simulink model "tadpole_dynamic_close_loop"  (R2019b)
settings: Solver=FixedStepAuto  StartTime=0.0  StopTime=sim_time  FixedStep=0.001  RelTol=1e-2
values from neighbouring files (symbols this model uses):
  C_alpha = 1000*ones(runcycle,1)    [rand_par.m]    (also in whole_par.m = 1000; whole_par_bias.m = 1000)
  C_beta = 50*ones(runcycle,1)    [rand_par.m]    (also in whole_par.m = 50; whole_par_bias.m = 50)
  Cd = 0.25*ones(runcycle,1)    [rand_par.m]    (also in whole_par.m = 0.25; whole_par_bias.m = 0.25)
  delta_fL = -1*ones(runcycle,1)    [rand_par.m]    (also in whole_par.m = -1; whole_par_bias.m = -1)
  delta_fR = 3.5*ones(runcycle,1)    [rand_par.m]    (also in whole_par.m = 3.5; whole_par_bias.m = 3.5)
  FA = 1*ones(runcycle,1)    [rand_par.m]    (also in whole_par.m = 1; whole_par_bias.m = 1)
  h = [ h(1:j-1) ; h(j+1:m)]    [UMDIRECT.m]    (also in whole_par.m = 0.4896; whole_par_bias.m = 0.4896)
  I_f_wheel = 0.3    [whole_par.m]    (also in whole_par_bias.m)
  I_r_wheel = 0.5    [whole_par.m]    (also in whole_par_bias.m)
  I_x = 12.1*ones(runcycle,1)    [rand_par.m]    (also in whole_par.m = 12.1; whole_par_bias.m = 12.1)
  I_y = 36.7*ones(runcycle,1)    [rand_par.m]    (also in whole_par.m = 36.7; whole_par_bias.m = 36.7)
  I_z = 50*DOE(:,2)    [rand_par.m]    (also in whole_par.m = 50; whole_par_bias.m = 60)
  k_z = 30000*ones(runcycle,1)    [rand_par.m]    (also in whole_par.m = 30000; whole_par_bias.m = 30000)
  l_1 = 0.724    [whole_par.m]    (also in whole_par_bias.m)
  l_2 = 0.719    [whole_par.m]    (also in whole_par_bias.m)
  m = m - 1    [UMDIRECT.m]    (also in rand_par.m = 48.3*DOE(:,1); whole_par.m = 48.3; whole_par_bias.m = 60)
  mu_dp = 0.8*ones(runcycle,1)    [rand_par.m]    (also in whole_par.m = 0.8; whole_par_bias.m = 0.8)
  mu_lp = 0.8*ones(runcycle,1)    [rand_par.m]    (also in whole_par.m = 0.8; whole_par_bias.m = 0.8)
  mu_rolling_1 = 0.009*ones(runcycle,1)    [rand_par.m]    (also in whole_par.m = 0.009; whole_par_bias.m = 0.009)
  mu_rolling_2 = 0.0005*ones(runcycle,1)    [rand_par.m]    (also in whole_par.m = 0.0005; whole_par_bias.m = 0.0005)
  R_0 = 0.335*ones(runcycle,1)    [rand_par.m]    (also in whole_par.m = 0.335; whole_par_bias.m = 0.335)
  rho = 1.225*ones(runcycle,1)    [rand_par.m]    (also in whole_par.m = 1.225; whole_par_bias.m = 1.225)
  SAP = 0.01*ones(runcycle,1)    [rand_par.m]    (also in whole_par.m = 0.01; whole_par_bias.m = 0.01)
  V_wind = 0*ones(runcycle,1)    [rand_par.m]    (also in whole_par.m = 0; whole_par_bias.m = 0)
  waypoint = [x' y']    [waypoints.m]
undefined symbols (not defined in the file or in its folder): DiscIntNeverNeededParam
libraries: simulink_extras x11, simulink x2, robotalgslib x1, mobileRoboticsLib x1
(part 2 of 4)

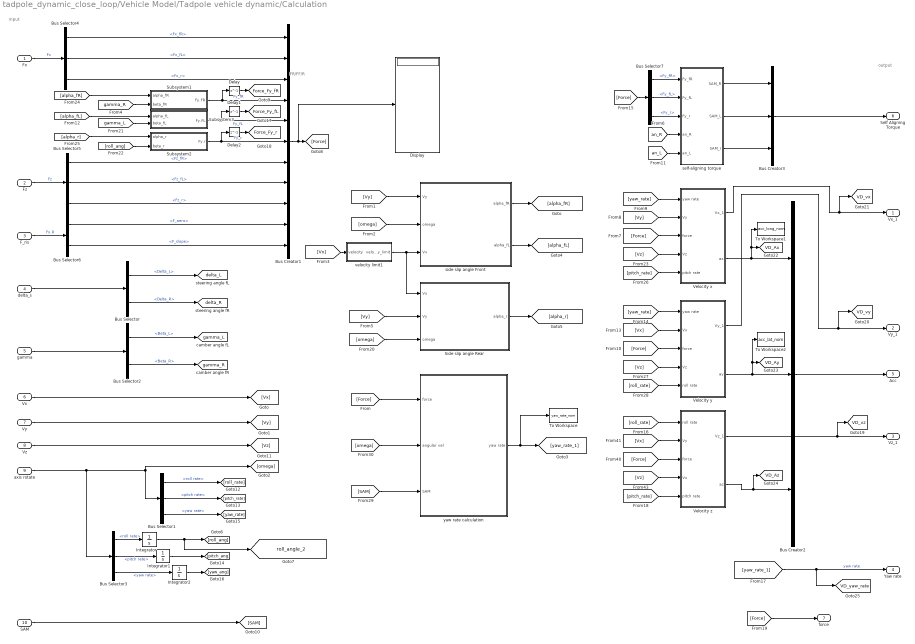
== system tadpole_dynamic_close_loop/Vehicle Model/Tadpole vehicle dynamic/Calculation ==
  note: input
  note: output
  note: FR/FF/R
  Fx : Inport
  Fz : Inport  Port=2
  F_ris : Inport  Port=3
  delta_s : Inport  Port=4
  gamma : Inport  Port=5
  Vx : Inport  Port=6
  Vy : Inport  Port=7
  Vz : Inport  Port=8
  axis rotate : Inport  Port=9
  SAM : Inport  Port=10
  Bus Creator1 : BusCreator  Inputs=11
  Bus Creator2 : BusCreator  Inputs=3
  Bus Creator3 : BusCreator  Inputs=3
  Bus Selector : BusSelector  OutputSignals=Delta_L,Delta_R
  Bus Selector1 : BusSelector  OutputSignals=roll rate,pitch rate,yaw rate
  Bus Selector2 : BusSelector  OutputSignals=Beta_L,Beta_R
  Bus Selector3 : BusSelector  OutputSignals=roll rate,pitch rate,yaw rate
  Bus Selector4 : BusSelector  OutputSignals=Fx_fR,Fx_fL,Fx_r
  Bus Selector5 : BusSelector  OutputSignals=Fz_fR,Fz_fL,Fz_r
  Bus Selector6 : BusSelector  OutputSignals=F_aero,F_slope
  Bus Selector7 : BusSelector  OutputSignals=Fy_fR,Fy_fL,Fy_r
  Delay : Delay  DelayLength=1
  Delay1 : Delay  DelayLength=1
  Delay2 : Delay  DelayLength=1
  Display : Display
  Integrator : Integrator
  Integrator1 : Integrator
  Integrator2 : Integrator
  Side slip angle Rear : Subsystem
  Subsystem1 : Subsystem
  Subsystem2 : Subsystem
  Subsystem3 : Subsystem
  To Workspace : ToWorkspace  VariableName=yaw_rate_nom  SaveFormat=Timeseries  SampleTime=-1
  To Workspace1 : ToWorkspace  VariableName=acc_long_nom  SaveFormat=Timeseries  SampleTime=-1
  To Workspace2 : ToWorkspace  VariableName=acc_lat_nom  SaveFormat=Timeseries  SampleTime=-1
  Velocity x : Subsystem
  Velocity y : Subsystem
  Velocity z : Subsystem
  self-aligning torque : Subsystem
  side slip angle Front : Subsystem
  velocity limit1 : Subsystem
  yaw rate calculation : Subsystem
  Vx_1 : Outport  VectorParamsAs1DForOutWhenUnconnected=off
  Vy_1 : Outport  Port=2  VectorParamsAs1DForOutWhenUnconnected=off
  Vz_1 : Outport  Port=3  VectorParamsAs1DForOutWhenUnconnected=off
  Yaw rate : Outport  Port=4  VectorParamsAs1DForOutWhenUnconnected=off
  Acc : Outport  Port=5  VectorParamsAs1DForOutWhenUnconnected=off
  Self Aligning Torque : Outport  Port=6  VectorParamsAs1DForOutWhenUnconnected=off
  force : Outport  Port=7  VectorParamsAs1DForOutWhenUnconnected=off
  tag scope: Force_Fy_fL=global, Force_Fy_fR=global, Force_Fy_r=global, VD_Ax=global, VD_Ay=global, VD_Az=global, VD_vx=global, VD_vy=global, VD_vz=global, VD_yaw_rate=global, delta_L=global, delta_R=global, gamma_L=global, gamma_R=global, roll_angle_2=global
  wires:
  delta_s/1 -> Bus Selector/1
  Bus Selector/1 -> [delta_L]  "<Delta_L>"
  Bus Selector/2 -> [delta_R]  "<Delta_R>"
  Vx/1 -> [Vx]
  Vy/1 -> [Vy]
  [Force] -> yaw rate calculation/1(force)
  yaw rate calculation/1(yaw rate) -> To Workspace/1, [yaw_rate_1]
  Bus Creator1/1 -> Display/1, [Force]
  [Vy] -> side slip angle Front/1(Vy)
  [omega] -> side slip angle Front/2(omega)
  [omega] -> Side slip angle Rear/3(omega)
  [Vy] -> Side slip angle Rear/2(Vy)
  side slip angle Front/1(alpha_fR) -> [alpha_fR]
  side slip angle Front/2(alpha_fL) -> [alpha_fL]
  Side slip angle Rear/1(alpha_r) -> [alpha_r]
  self-aligning torque/1(SAM_R) -> Bus Creator3/1
  self-aligning torque/2(SAM_L) -> Bus Creator3/2
  [Vx] -> velocity limit1/1("velocity ")
  velocity limit1/1("velocity_limit ") -> Side slip angle Rear/1(Vx), side slip angle Front/3(Vx)
  [yaw_rate] -> Velocity x/1(yaw rate)
  [Vy] -> Velocity x/2(Vy)
  [Force] -> Velocity x/3("force ")
  Velocity x/1(Vx_1) -> [VD_vx], Vx_1/1
  Velocity x/2(ax) -> To Workspace1/1, [VD_Ax], Bus Creator2/1
  [Force] -> Velocity y/3("force ")
  Velocity y/1(Vy_1) -> [VD_vy], Vy_1/1
  [yaw_rate] -> Velocity y/1(yaw rate)
  [Vx] -> Velocity y/2(Vx)
  Velocity y/2(ay) -> To Workspace2/1, [VD_Ay], Bus Creator2/2
  [yaw_rate_1] -> [VD_yaw_rate], Yaw rate/1  "yaw rate"
  SAM/1 -> [SAM]
  [Vz] -> Velocity x/4(Vz)
  [pitch_rate] -> Velocity x/5(pitch rate)
  Vz/1 -> [Vz]
  Bus Selector1/1 -> [roll_rate]  "<roll rate>"
  Bus Selector1/2 -> [pitch_rate]  "<pitch rate>"
  Bus Selector1/3 -> [yaw_rate]  "<yaw rate>"
  [Vz] -> Velocity y/4(Vz)
  [roll_rate] -> Velocity y/5(roll rate)
  [SAM] -> yaw rate calculation/3(SAM)
  [omega] -> yaw rate calculation/2(angular vel)
  self-aligning torque/3(SAM_r) -> Bus Creator3/3
  Velocity z/1(Vz_1) -> [VD_vz], Vz_1/1
  [Vx] -> Velocity z/2(Vy)
  [pitch_rate] -> Velocity z/5(pitch rate)
  [roll_rate] -> Velocity z/1(roll rate)
  [Force] -> Velocity z/3("force ")
  Velocity z/2(az) -> [VD_Az], Bus Creator2/3
  [Vz] -> Velocity z/4(Vx)
  Bus Creator2/1 -> Acc/1
  Bus Creator3/1 -> Self Aligning Torque/1
  gamma/1 -> Bus Selector2/1
  Bus Selector2/1 -> [gamma_L]  "<Beta_L>"
  Bus Selector2/2 -> [gamma_R]  "<Beta_R>"
  Bus Selector3/3 -> Integrator2/1  "<yaw rate>"
  Bus Selector3/2 -> Integrator1/1  "<pitch rate>"
  Bus Selector3/1 -> Integrator/1  "<roll rate>"
  axis rotate/1 -> Bus Selector3/1, [omega], Bus Selector1/1
  Integrator/1 -> [roll_angle_2], [roll_ang]
  Integrator1/1 -> [pitch_ang]
  Integrator2/1 -> [yaw_ang]
  Fx/1 -> Bus Selector4/1  "Fx"
  Bus Selector4/1 -> Bus Creator1/1  "<Fx_fR>"
  Bus Selector4/2 -> Bus Creator1/2  "<Fx_fL>"
  Bus Selector4/3 -> Bus Creator1/3  "<Fx_r>"
  [gamma_L] -> Subsystem3/2(beta_fL)
  [alpha_fR] -> Subsystem1/1(alpha_fR)
  [gamma_R] -> Subsystem1/2(beta_fR)
  [alpha_fL] -> Subsystem3/1(alpha_fL)
  [roll_ang] -> Subsystem2/2(beta_r)
  [alpha_r] -> Subsystem2/1(alpha_r)
  Subsystem1/1(Fy.FR) -> Bus Creator1/4, Delay/1  "Fy_fR"
  Subsystem3/1(Fy.FL) -> Delay1/1, Bus Creator1/5  "Fy_fL"
  Subsystem2/1(Fy.r) -> Delay2/1, Bus Creator1/6  "Fy_r"
  Fz/1 -> Bus Selector5/1  "Fz"
  Bus Selector5/2 -> Bus Creator1/8  "<Fz_fL>"
  Bus Selector5/1 -> Bus Creator1/7  "<Fz_fR>"
  Bus Selector5/3 -> Bus Creator1/9  "<Fz_r>"
  F_ris/1 -> Bus Selector6/1  "Fx.R"
  Bus Selector6/1 -> Bus Creator1/10  "<F_aero>"
  Bus Selector6/2 -> Bus Creator1/11  "<F_slope>"
  [Force] -> force/1
  [an_R] -> self-aligning torque/4(an_R)
  [an_L] -> self-aligning torque/5(an_L)
  [Force] -> Bus Selector7/1
  Bus Selector7/1 -> self-aligning torque/1(Fy_fR)  "<Fy_fR>"
  Bus Selector7/2 -> self-aligning torque/2(Fy_fL)  "<Fy_fL>"
  Bus Selector7/3 -> self-aligning torque/3(Fy_r)  "<Fy_r>"
  Delay/1 -> [Force_Fy_fR]
  Delay1/1 -> [Force_Fy_fL]
  Delay2/1 -> [Force_Fy_r]

== system tadpole_dynamic_close_loop/Vehicle Model/Tadpole vehicle dynamic/Velocity ==
  Vx : Inport
  Vy : Inport  Port=2
  Add : Sum
  Power : Math  Operator=pow  SaturateOnIntegerOverflow=on
  Power1 : Math  Operator=pow  SaturateOnIntegerOverflow=on
  Sqrt : Sqrt  SaturateOnIntegerOverflow=on
  power : Constant  Value=2
  power 2 : Constant  Value=2
  absolute V : Outport  VectorParamsAs1DForOutWhenUnconnected=off
  wires:
  Power1/1 -> Add/2  "Vy^2"
  power/1 -> Power1/2
  Power/1 -> Add/1  "Vx^2"
  power 2/1 -> Power/2
  Vx/1 -> Power/1
  Vy/1 -> Power1/1
  Add/1 -> Sqrt/1
  Sqrt/1 -> absolute V/1

== system tadpole_dynamic_close_loop/Vehicle Model/Tadpole vehicle dynamic/local to global ==
  Vy : Inport
  yaw rate : Inport  Port=2
  Vx : Inport  Port=3
  Add : Sum
  Add1 : Sum
  Gain : Gain  Gain=-1
  Integrator : Integrator
  Multiply{,1..3} (4 alike) : Product
  Sin : Trigonometry
  Sin1 : Trigonometry  Operator=cos
  absolute x dot : Outport  VectorParamsAs1DForOutWhenUnconnected=off
  absolute y dot : Outport  Port=2  VectorParamsAs1DForOutWhenUnconnected=off
  tag scope: VD_yaw_angle=global
  wires:
  Gain/1 -> Add/2
  Vx/1 -> Multiply/2, Multiply2/2
  Multiply1/1 -> Gain/1
  Sin/1 -> Multiply2/1, Multiply1/1
  Multiply3/1 -> Add1/2
  Integrator/1 -> [VD_yaw_angle], [A]
  Sin1/1 -> Multiply3/1, Multiply/1
  Multiply/1 -> Add/1
  Vy/1 -> Multiply3/2, Multiply1/2
  Add/1 -> absolute x dot/1  "absolute x dot"
  [A] -> Sin1/1, Sin/1
  Multiply2/1 -> Add1/1
  Add1/1 -> absolute y dot/1
  yaw rate/1 -> Integrator/1

== system tadpole_dynamic_close_loop/Vehicle Model/resistance calculation/Aerodynamic Drag Force ==
  Vx : Inport
  Add : Sum
  Air density : Constant  Value=rho
  Constant : Constant  Value=V_wind
  Constant5 : Constant  Value=0.5
  Constant6 : Constant  Value=2
  "Drag coefficient " : Constant  Value=Cd
  Front Area : Constant  Value=FA
  Gain : Gain  Gain=-1
  Math Function : Math  Operator=pow  SaturateOnIntegerOverflow=on
  Product1 : Product  Inputs=6
  Sign : Signum
  F_aero : Outport  VectorParamsAs1DForOutWhenUnconnected=off
  wires:
  Add/1 -> Math Function/1, Sign/1
  Constant6/1 -> Math Function/2
  "Drag coefficient "/1 -> Product1/3
  Product1/1 -> F_aero/1
  Math Function/1 -> Product1/5
  Constant5/1 -> Product1/1
  Air density/1 -> Product1/4
  Front Area/1 -> Product1/2
  Sign/1 -> Gain/1
  Gain/1 -> Product1/6
  Vx/1 -> Add/1
  Constant/1 -> Add/2

== system tadpole_dynamic_close_loop/Vehicle Model/resistance calculation/Rear Traction add up ==
  break : Inport
  motor : Inport  Port=2
  V sign : Inport  Port=3
  Abs : Abs
  Abs1 : Abs
  Fm<0 : Subsystem  TreatAsAtomicUnit=on
  Fm>=0 : Subsystem  TreatAsAtomicUnit=on
  If (check motor sign) : If  IfExpression=u1 >= 0
  Merge : Merge
  Scope : Scope
  Rear Traction : Outport  VectorParamsAs1DForOutWhenUnconnected=off
  wires:
  Abs/1 -> Fm<0/1(|break|), Scope/1, Fm>=0/1(|break|)  "break"
  motor/1 -> If (check motor sign)/1, Abs1/1
  Abs1/1 -> Fm<0/2(|motor|), Fm>=0/2(|motor|)  "motor"
  break/1 -> Abs/1
  If (check motor sign)/1 -> Fm>=0/Action
  If (check motor sign)/2 -> Fm<0/Action
  Fm>=0/1(Out1) -> Merge/1
  Fm<0/1(Out1) -> Merge/2
  Merge/1 -> Rear Traction/1
  V sign/1 -> Fm<0/3("velocity sign "), Fm>=0/3("velocity sign ")  "velocity sign"

== system tadpole_dynamic_close_loop/Vehicle Model/resistance calculation/Rolling Resistance Force Front L ==
  Fz_fL : Inport
  Vx : Inport  Port=2
  Vy : Inport  Port=3
  yaw rate : Inport  Port=4
  Delta_L : Inport  Port=5
  Gain : Gain  Gain=-1
  Multiply : Product  Inputs=3
  Scope : Scope
  Sign : Signum
  Subsystem : Subsystem
  mu(v) : Subsystem
  Frr_fL : Outport  VectorParamsAs1DForOutWhenUnconnected=off
  wires:
  Fz_fL/1 -> Multiply/1  "Fzr"
  Subsystem/1(Vx_Wheel) -> mu(v)/1(Vx), Sign/1
  Gain/1 -> Multiply/3
  mu(v)/1(mu_rolling) -> Multiply/2
  Sign/1 -> Gain/1
  Vx/1 -> Subsystem/1(Vx)
  Vy/1 -> Subsystem/2(Vy)
  yaw rate/1 -> Subsystem/3(yaw rate)
  Delta_L/1 -> Subsystem/4(Delta_L)
  Multiply/1 -> Scope/1, Frr_fL/1

== system tadpole_dynamic_close_loop/Vehicle Model/resistance calculation/Rolling Resistance Force Front R ==
  Fz_fR : Inport
  Vx : Inport  Port=2
  Vy : Inport  Port=3
  yaw rate : Inport  Port=4
  Delta_R : Inport  Port=5
  Gain : Gain  Gain=-1
  Multiply : Product  Inputs=3
  Sign : Signum
  Subsystem : Subsystem
  mu(v) : Subsystem
  Frr_fR : Outport  VectorParamsAs1DForOutWhenUnconnected=off
  wires:
  Fz_fR/1 -> Multiply/1  "Fzr"
  Subsystem/1(Vx_Wheel) -> mu(v)/1(Vx), Sign/1
  Gain/1 -> Multiply/3
  mu(v)/1(mu_rolling) -> Multiply/2
  Sign/1 -> Gain/1
  Vx/1 -> Subsystem/1(Vx)
  Vy/1 -> Subsystem/2(Vy)
  yaw rate/1 -> Subsystem/3(yaw rate)
  Delta_R/1 -> Subsystem/4(Delta_R)
  Multiply/1 -> Frr_fR/1

== system tadpole_dynamic_close_loop/Vehicle Model/resistance calculation/Rolling Resistance Force Rear ==
  Fz_r : Inport
  velocity sign : Inport  Port=2
  Vx : Inport  Port=3
  Gain : Gain  Gain=-1
  Multiply : Product  Inputs=3
  mu(v) : Subsystem
  Frr : Outport  VectorParamsAs1DForOutWhenUnconnected=off
  wires:
  Multiply/1 -> Frr/1
  Fz_r/1 -> Multiply/1  "Fzr"
  velocity sign/1 -> Gain/1
  Gain/1 -> Multiply/3
  mu(v)/1(mu_rolling) -> Multiply/2
  Vx/1 -> mu(v)/1(Vx)

== system tadpole_dynamic_close_loop/Vehicle Model/resistance calculation/linear slip cal.  ==
  rear traction : Inport
  rear normal force : Inport  Port=2
  Display : Display
  Gain2 : Gain  Gain=-1
  MinMax : MinMax  Inputs=2
  MinMax2 : MinMax  Function=max  Inputs=2
  Product : Product
  max. long. friction coefficient : Constant  Value=mu_dp
  slip recgonition : Subsystem
  "Rear Traction " : Outport  VectorParamsAs1DForOutWhenUnconnected=off
  wires:
  Gain2/1 -> MinMax2/2
  Product/1 -> Gain2/1, slip recgonition/1(In2), MinMax/1
  MinMax/1 -> slip recgonition/2(In3), Display/1, MinMax2/1
  MinMax2/1 -> "Rear Traction "/1
  rear traction/1 -> MinMax/2
  rear normal force/1 -> Product/2
  max. long. friction coefficient/1 -> Product/1

== system tadpole_dynamic_close_loop/Vehicle Model/resistance calculation/slope  ==
  Slope : Inport
  Degrees to Radians : simulink_extras/Transformations/Degrees to Radians
  Gain : Gain  Gain=-1
  Gain1 : Gain  Gain=9.81
  Product : Product
  Sin : Trigonometry
  mass : Constant  Value=m
  F_slope : Outport  VectorParamsAs1DForOutWhenUnconnected=off
  wires:
  Gain1/1 -> Product/1
  Sin/1 -> Product/2
  Slope/1 -> Degrees to Radians/1
  Product/1 -> Gain/1  "Slope"
  Gain/1 -> F_slope/1
  mass/1 -> Gain1/1
  Degrees to Radians/1 -> Sin/1

== system tadpole_dynamic_close_loop/Vehicle Model/resistance calculation/torque to force ==
  traction torque : Inport
  rear normal force : Inport  Port=2
  Add : Sum  Inputs=+-
  Divide1 : Product  Inputs=*/
  Divide2 : Product  Inputs=*/
  Initial wheel radius : Constant  Value=R_0
  tire vertical stiffness : Constant  Value=k_z
  rear traction F : Outport  VectorParamsAs1DForOutWhenUnconnected=off
  tag scope: R_h=global
  wires:
  traction torque/1 -> Divide1/1
  Divide1/1 -> rear traction F/1
  tire vertical stiffness/1 -> Divide2/2
  rear normal force/1 -> Divide2/1
  Divide2/1 -> Add/2
  Initial wheel radius/1 -> Add/1
  Add/1 -> [R_h], Divide1/2  "effective radius"

== system tadpole_dynamic_close_loop/Vehicle Model/resistance calculation/velocity limit x ==
  "velocity " : Inport
  If Action Subsystem2 : Subsystem  TreatAsAtomicUnit=on
  If Action Subsystem3 : Subsystem  TreatAsAtomicUnit=on
  If1 : If  IfExpression=u1>0
  Merge : Merge
  "velocity_limit " : Outport  VectorParamsAs1DForOutWhenUnconnected=off
  wires:
  Merge/1 -> "velocity_limit "/1
  "velocity "/1 -> If Action Subsystem3/1(In1), If Action Subsystem2/1(In1), If1/1
  If1/1 -> If Action Subsystem2/Action
  If1/2 -> If Action Subsystem3/Action
  If Action Subsystem2/1(Out1) -> Merge/1
  If Action Subsystem3/1(Out1) -> Merge/2

== system tadpole_dynamic_close_loop/Vehicle Model/resistance calculation/velocity limit y ==
  "velocity " : Inport
  If Action Subsystem2 : Subsystem  TreatAsAtomicUnit=on
  If Action Subsystem3 : Subsystem  TreatAsAtomicUnit=on
  If1 : If  IfExpression=u1>0
  Merge : Merge
  "velocity_limit " : Outport  VectorParamsAs1DForOutWhenUnconnected=off
  wires:
  Merge/1 -> "velocity_limit "/1
  "velocity "/1 -> If Action Subsystem3/1(In1), If Action Subsystem2/1(In1), If1/1
  If1/1 -> If Action Subsystem2/Action
  If1/2 -> If Action Subsystem3/Action
  If Action Subsystem2/1(Out1) -> Merge/1
  If Action Subsystem3/1(Out1) -> Merge/2

== system tadpole_dynamic_close_loop/Vehicle Model/Tadpole vehicle dynamic/Calculation/Side slip angle Rear ==
  Vx : Inport
  Vy : Inport  Port=2
  omega : Inport  Port=3
  Add : Sum  Inputs=+-
  Atan1 : Trigonometry  Operator=atan
  Bus Selector : BusSelector  OutputSignals=yaw rate
  Constant : Constant
  Constant1 : Constant
  Constant4 : Constant  Value=0
  Constant7 : Constant  Value=l_2
  Divide4 : Product  Inputs=*/
  Minus1 : Sum  Inputs=+-
  Multiply1 : Product
  Product : Product
  Radians to Degrees1 : simulink_extras/Transformations/Radians to Degrees
  Switch : Switch  Criteria=u2 ~= 0
  Switch1 : Switch  Criteria=u2 ~= 0
  delta_rear : Constant  Value=0
  velocity limit1 : Subsystem
  alpha_r : Outport  VectorParamsAs1DForOutWhenUnconnected=off
  tag scope: VD_Vy_r=global, VD_alpha_r=global
  wires:
  Switch/1 -> Divide4/2
  Constant/1 -> Switch/3
  Divide4/1 -> Atan1/1
  Add/1 -> Product/1  "alpha_r"
  Constant7/1 -> Multiply1/1
  Vy/1 -> Minus1/1
  Atan1/1 -> Add/2
  Minus1/1 -> [VD_Vy_r], Divide4/1
  Multiply1/1 -> Minus1/2
  [yaw_rate] -> Multiply1/2
  omega/1 -> Bus Selector/1
  Bus Selector/1 -> [yaw_rate]  "<yaw rate>"
  delta_rear/1 -> Add/1
  Constant4/1 -> Switch1/3
  Vx/1 -> velocity limit1/1("velocity "), Switch/1, Switch/2
  Switch1/1 -> Product/2
  Constant1/1 -> Switch1/1
  velocity limit1/1("velocity_limit ") -> Switch1/2
  Product/1 -> Radians to Degrees1/1, alpha_r/1
  Radians to Degrees1/1 -> [VD_alpha_r]

== system tadpole_dynamic_close_loop/Vehicle Model/Tadpole vehicle dynamic/Calculation/Subsystem1 ==
  alpha_fR : Inport
  beta_fR : Inport  Port=2
  Add : Sum
  Bus Selector : BusSelector  OutputSignals=Vx
  Gain : Gain  Gain=C_alpha
  Gain1 : Gain  Gain=C_beta
  IC : InitialCondition  Value=0
  Product : Product
  Scope : Scope  NumInputPorts=3
  Sign : Signum
  Subsystem : Subsystem
  velocity limit : Subsystem
  Fy.FR : Outport  VectorParamsAs1DForOutWhenUnconnected=off
  tag scope: Force_Fy_fR_camber=global, Force_Fy_fR_sideslip=global
  wires:
  Gain/1 -> [Force_Fy_fR_sideslip], Scope/1, Add/1  "Fy.FR sideslip"
  alpha_fR/1 -> Gain/1
  Add/1 -> Product/1
  Gain1/1 -> [Force_Fy_fR_camber], Scope/2, Add/2  "Fy.FR camber"
  beta_fR/1 -> Gain1/1
  [V] -> Bus Selector/1
  velocity limit/1("velocity_limit ") -> Sign/1
  Sign/1 -> Scope/3, Product/2
  Product/1 -> Subsystem/1(Fy_fR)
  Bus Selector/1 -> velocity limit/1("velocity ")  "<Vx>"
  Subsystem/1(Lateral force fR) -> IC/1
  IC/1 -> Fy.FR/1

== system tadpole_dynamic_close_loop/Vehicle Model/Tadpole vehicle dynamic/Calculation/Subsystem2 ==
  alpha_r : Inport
  beta_r : Inport  Port=2
  Add : Sum
  Bus Selector : BusSelector  OutputSignals=Vx
  Gain2 : Gain  Gain=C_alpha
  Gain3 : Gain  Gain=C_beta
  Product : Product
  Sign : Signum
  Subsystem : Subsystem
  velocity limit : Subsystem
  Fy.r : Outport  VectorParamsAs1DForOutWhenUnconnected=off
  tag scope: Force_Fy_r_camber=global, Force_Fy_r_sideslip=global
  wires:
  beta_r/1 -> Gain3/1
  Gain3/1 -> [Force_Fy_r_camber], Add/2  "Fy.r camber"
  alpha_r/1 -> Gain2/1
  Add/1 -> Product/1
  Gain2/1 -> [Force_Fy_r_sideslip], Add/1  "Fy.r sideslip"
  velocity limit/1("velocity_limit ") -> Sign/1
  Sign/1 -> Product/2
  Product/1 -> Subsystem/1(Fy_fL)
  [V] -> Bus Selector/1
  Bus Selector/1 -> velocity limit/1("velocity ")  "<Vx>"
  Subsystem/1(Lateral Force r) -> Fy.r/1

== system tadpole_dynamic_close_loop/Vehicle Model/Tadpole vehicle dynamic/Calculation/Subsystem3 ==
  alpha_fL : Inport
  beta_fL : Inport  Port=2
  Add : Sum
  Bus Selector : BusSelector  OutputSignals=Vx
  Gain1 : Gain  Gain=C_alpha
  Gain2 : Gain  Gain=C_beta
  Product : Product
  Sign : Signum
  Subsystem : Subsystem
  velocity limit : Subsystem
  Fy.FL : Outport  VectorParamsAs1DForOutWhenUnconnected=off
  tag scope: Force_Fy_fL_camber=global, Force_Fy_fL_sideslip=global
  wires:
  Add/1 -> Product/1
  alpha_fL/1 -> Gain1/1
  beta_fL/1 -> Gain2/1
  Gain1/1 -> [Force_Fy_fL_sideslip], Add/1  "Fy.FL sideslip"
  Gain2/1 -> [Force_Fy_fL_camber], Add/2  "Fy.FL camber"
  velocity limit/1("velocity_limit ") -> Sign/1
  Sign/1 -> Product/2
  Product/1 -> Subsystem/1(Fy_fL)
  [V] -> Bus Selector/1
  Bus Selector/1 -> velocity limit/1("velocity ")  "<Vx>"
  Subsystem/1(Lateral Force fL) -> Fy.FL/1

== system tadpole_dynamic_close_loop/Vehicle Model/Tadpole vehicle dynamic/Calculation/Velocity x ==
  note: Vx'
  note: Equation of Vx
  note: Vx
  yaw rate : Inport
  Vy : Inport  Port=2
  "force " : Inport  Port=3
  Vz : Inport  Port=4
  pitch rate : Inport  Port=5
  Add : Sum  Inputs=-++
  Bus Selector : BusSelector  OutputSignals=Fx_fR,Fx_fL,Fy_fR,Fy_fL,Fx_r
  Divide : Product  Inputs=*/
  Equivalent mass : Subsystem
  Gain : Gain  Gain=-1
  Gain1 : Gain  Gain=-1
  Integrator : Integrator
  Multiply{1..4} (4 alike) : Product
  Product : Product
  Product1 : Product
  Sin1 : Trigonometry  Operator=cos
  Sin2 : Trigonometry  Operator=cos
  Sin3 : Trigonometry
  Sin4 : Trigonometry
  Sum1 : Sum  Inputs=+++++
  Vx_1 : Outport  VectorParamsAs1DForOutWhenUnconnected=off
  ax : Outport  Port=2  VectorParamsAs1DForOutWhenUnconnected=off
  tag scope: Force_Fx=global
  wires:
  Product/1 -> Add/2
  yaw rate/1 -> Product/2
  Vy/1 -> Product/1
  Integrator/1 -> Vx_1/1
  Add/1 -> ax/1, Integrator/1
  "force "/1 -> Bus Selector/1
  Bus Selector/1 -> Multiply2/2  "<Fx_fR>"
  Sin2/1 -> Multiply2/1
  [delta_R] -> Sin2/1
  Sin1/1 -> Multiply1/1
  [delta_L] -> Sin1/1
  Bus Selector/2 -> Multiply1/2  "<Fx_fL>"
  [delta_R] -> Sin3/1
  Sin3/1 -> Multiply3/1
  Bus Selector/3 -> Gain/1  "<Fy_fR>"
  Gain/1 -> Multiply3/2
  Sin4/1 -> Multiply4/1
  [delta_L] -> Sin4/1
  Gain1/1 -> Multiply4/2
  Bus Selector/4 -> Gain1/1  "<Fy_fL>"
  Multiply2/1 -> Sum1/1
  Multiply1/1 -> Sum1/2
  Multiply3/1 -> Sum1/3
  Multiply4/1 -> Sum1/4
  Bus Selector/5 -> Sum1/5  "<Fx_r>"
  Sum1/1 -> [Force_Fx], Divide/1
  Divide/1 -> Add/3
  Vz/1 -> Product1/1
  pitch rate/1 -> Product1/2
  Product1/1 -> Add/1
  Equivalent mass/1(Mass_eq) -> Divide/2

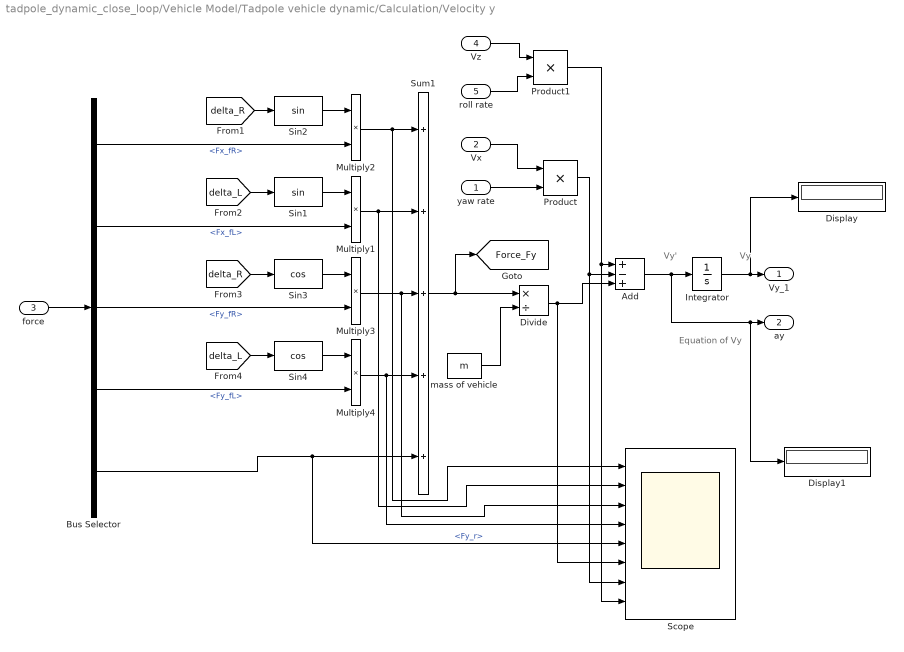
== system tadpole_dynamic_close_loop/Vehicle Model/Tadpole vehicle dynamic/Calculation/Velocity y ==
  note: Vy'
  note: Equation of Vy
  note: Vy
  yaw rate : Inport
  Vx : Inport  Port=2
  "force " : Inport  Port=3
  Vz : Inport  Port=4
  roll rate : Inport  Port=5
  Add : Sum  Inputs=+-+
  Bus Selector : BusSelector  OutputSignals=Fx_fR,Fx_fL,Fy_fR,Fy_fL,Fy_r
  Display : Display
  Display1 : Display
  Divide : Product  Inputs=*/
  Integrator : Integrator
  Multiply{1..4} (4 alike) : Product
  Product : Product
  Product1 : Product
  Scope : Scope  NumInputPorts=8
  Sin1 : Trigonometry
  Sin2 : Trigonometry
  Sin3 : Trigonometry  Operator=cos
  Sin4 : Trigonometry  Operator=cos
  Sum1 : Sum  Inputs=+++++
  mass of vehicle : Constant  Value=m
  Vy_1 : Outport  VectorParamsAs1DForOutWhenUnconnected=off
  ay : Outport  Port=2  VectorParamsAs1DForOutWhenUnconnected=off
  tag scope: Force_Fy=global
  wires:
  Product/1 -> Scope/7, Add/2
  yaw rate/1 -> Product/2
  Vx/1 -> Product/1
  Integrator/1 -> Display/1, Vy_1/1
  Add/1 -> Display1/1, ay/1, Integrator/1
  "force "/1 -> Bus Selector/1
  Bus Selector/1 -> Multiply2/2  "<Fx_fR>"
  Sin2/1 -> Multiply2/1
  [delta_R] -> Sin2/1
  Sin1/1 -> Multiply1/1
  [delta_L] -> Sin1/1
  Bus Selector/2 -> Multiply1/2  "<Fx_fL>"
  [delta_R] -> Sin3/1
  Sin3/1 -> Multiply3/1
  Bus Selector/3 -> Multiply3/2  "<Fy_fR>"
  Sin4/1 -> Multiply4/1
  [delta_L] -> Sin4/1
  Bus Selector/4 -> Multiply4/2  "<Fy_fL>"
  Multiply2/1 -> Scope/1, Sum1/1
  Multiply1/1 -> Scope/2, Sum1/2
  Multiply3/1 -> Scope/3, Sum1/3
  Multiply4/1 -> Scope/4, Sum1/4
  Bus Selector/5 -> Scope/5, Sum1/5  "<Fy_r>"
  Sum1/1 -> [Force_Fy], Divide/1
  Divide/1 -> Scope/6, Add/3
  mass of vehicle/1 -> Divide/2
  Product1/1 -> Scope/8, Add/1
  roll rate/1 -> Product1/2
  Vz/1 -> Product1/1

== system tadpole_dynamic_close_loop/Vehicle Model/Tadpole vehicle dynamic/Calculation/Velocity z ==
  note: Vz'
  note: Equation of Vz
  note: Vz
  roll rate : Inport
  Vy : Inport  Port=2
  "force " : Inport  Port=3
  Vx : Inport  Port=4
  pitch rate : Inport  Port=5
  Add : Sum  Inputs=+-+
  Bus Selector : BusSelector  OutputSignals=Fz_fL,Fz_fR,Fz_r
  Display : Display
  Display1 : Display
  Display2 : Display
  Divide : Product  Inputs=*/
  G : Gain  Gain=9.81
  Integrator : Integrator
  Product : Product
  Product1 : Product
  Sum1 : Sum  Inputs=+++-
  mass of vehicle : Constant  Value=m
  Vz_1 : Outport  VectorParamsAs1DForOutWhenUnconnected=off
  az : Outport  Port=2  VectorParamsAs1DForOutWhenUnconnected=off
  wires:
  Product/1 -> Display1/1, Add/2
  roll rate/1 -> Display2/1, Product/2
  Vy/1 -> Product/1
  Integrator/1 -> Vz_1/1
  "force "/1 -> Bus Selector/1
  Sum1/1 -> Divide/1
  Divide/1 -> Add/3
  mass of vehicle/1 -> G/1, Divide/2
  Product1/1 -> Display/1, Add/1
  pitch rate/1 -> Product1/2
  Vx/1 -> Product1/1
  Bus Selector/1 -> [Fz_fl]  "<Fz_fL>"
  Bus Selector/2 -> [Fz_fr]  "<Fz_fR>"
  Bus Selector/3 -> [Fz_r]  "<Fz_r>"
  [Fz_fl] -> Sum1/1
  [Fz_fr] -> Sum1/2
  [Fz_r] -> Sum1/3
  G/1 -> Sum1/4
  Add/1 -> Integrator/1, az/1

== system tadpole_dynamic_close_loop/Vehicle Model/Tadpole vehicle dynamic/Calculation/self-aligning torque ==
  Fy_fR : Inport
  Fy_fL : Inport  Port=2
  Fy_r : Inport  Port=3
  an_R : Inport  Port=4
  an_L : Inport  Port=5
  Add : Sum
  Add1 : Sum
  Constant1 : Constant  Value=SAP
  Constant2 : Constant  Value=SAP
  Gain1 : Gain  Gain=-1
  Gain2 : Gain  Gain=0
  Gain3 : Gain  Gain=-1
  Product{,1..3} (4 alike) : Product
  SAM_R : Outport  VectorParamsAs1DForOutWhenUnconnected=off
  SAM_L : Outport  Port=2  VectorParamsAs1DForOutWhenUnconnected=off
  SAM_r : Outport  Port=3  VectorParamsAs1DForOutWhenUnconnected=off
  tag scope: Force_SAM_L=global, Force_SAM_R=global
  wires:
  an_R/1 -> Product/1
  Fy_fR/1 -> Gain3/1
  Fy_fL/1 -> Gain1/1
  an_L/1 -> Product1/1
  Gain2/1 -> SAM_r/1  "Self aligning moment r"
  Fy_r/1 -> Gain2/1
  Gain1/1 -> Product2/2, Product1/2
  Product1/1 -> Add/1
  Add/1 -> [Force_SAM_L], SAM_L/1  "Self aligning moment L"
  Constant1/1 -> Product2/1
  Product2/1 -> Add/2
  Gain3/1 -> Product3/2, Product/2
  Constant2/1 -> Product3/1
  Product3/1 -> Add1/2
  Add1/1 -> [Force_SAM_R], SAM_R/1  "Self aligning moment R"
  Product/1 -> Add1/1

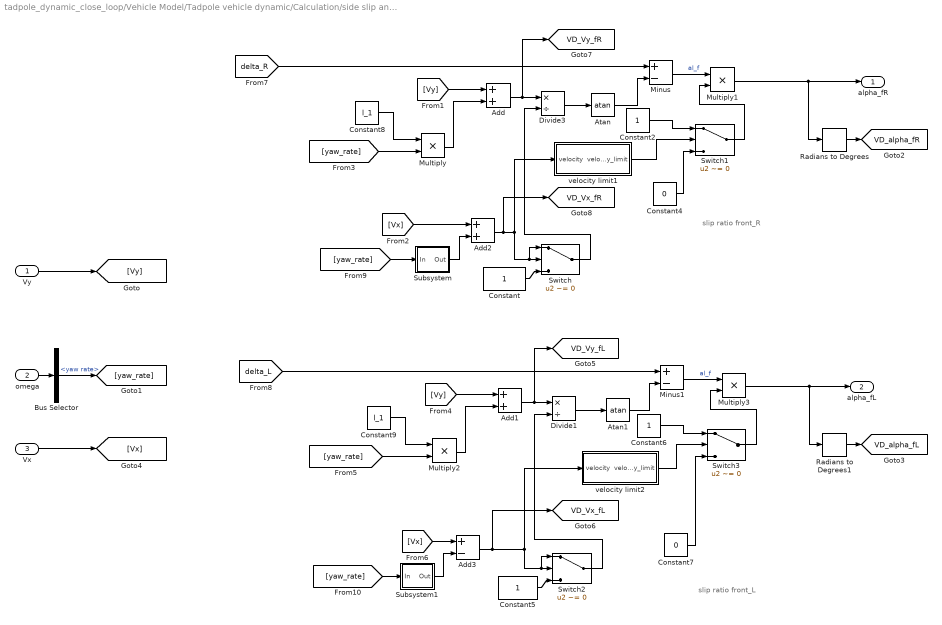
== system tadpole_dynamic_close_loop/Vehicle Model/Tadpole vehicle dynamic/Calculation/side slip angle Front ==
  note: slip ratio front_L
  note: slip ratio front_R
  Vy : Inport
  omega : Inport  Port=2
  Vx : Inport  Port=3
  Add : Sum
  Add1 : Sum
  Add2 : Sum
  Add3 : Sum  Inputs=+-
  Atan : Trigonometry  Operator=atan
  Atan1 : Trigonometry  Operator=atan
  Bus Selector : BusSelector  OutputSignals=yaw rate
  Constant{,2,5..6} (4 alike) : Constant
  Constant4 : Constant  Value=0
  Constant7 : Constant  Value=0
  Constant8 : Constant  Value=l_1
  Constant9 : Constant  Value=l_1
  Divide1 : Product  Inputs=*/
  Divide3 : Product  Inputs=*/
  Minus : Sum  Inputs=+-
  Minus1 : Sum  Inputs=+-
  Multiply{,1..3} (4 alike) : Product
  Radians to Degrees : simulink_extras/Transformations/Radians to Degrees
  Radians to Degrees1 : simulink_extras/Transformations/Radians to Degrees
  Subsystem : Subsystem
  Subsystem1 : Subsystem
  Switch{,1..3} (4 alike) : Switch  Criteria=u2 ~= 0
  velocity limit1 : Subsystem
  velocity limit2 : Subsystem
  alpha_fR : Outport  VectorParamsAs1DForOutWhenUnconnected=off
  alpha_fL : Outport  Port=2  VectorParamsAs1DForOutWhenUnconnected=off
  tag scope: VD_Vx_fL=global, VD_Vx_fR=global, VD_Vy_fL=global, VD_Vy_fR=global, VD_alpha_fL=global, VD_alpha_fR=global
  wires:
  Add3/1 -> [VD_Vx_fL], velocity limit2/1("velocity "), Switch2/2, Switch2/1
  Constant/1 -> Switch/3
  Atan1/1 -> Minus1/2
  Multiply1/1 -> Radians to Degrees/1, alpha_fR/1
  Constant9/1 -> Multiply2/1
  Vy/1 -> [Vy]
  Minus1/1 -> Multiply3/1  "al_f"
  Constant6/1 -> Switch3/1
  Constant8/1 -> Multiply/1
  [Vy] -> Add1/1
  Multiply/1 -> Add/2
  Add2/1 -> [VD_Vx_fR], velocity limit1/1("velocity "), Switch/1, Switch/2
  [yaw_rate] -> Multiply/2
  Switch2/1 -> Divide1/2
  Switch1/1 -> Multiply1/2
  Divide1/1 -> Atan1/1
  Constant2/1 -> Switch1/1
  Add1/1 -> [VD_Vy_fL], Divide1/1
  Add/1 -> [VD_Vy_fR], Divide3/1
  Constant4/1 -> Switch1/3
  Minus/1 -> Multiply1/1  "al_f"
  Constant7/1 -> Switch3/3
  Divide3/1 -> Atan/1
  Switch3/1 -> Multiply3/2
  Vx/1 -> [Vx]
  Atan/1 -> Minus/2
  [yaw_rate] -> Multiply2/2
  Switch/1 -> Divide3/2
  Constant5/1 -> Switch2/3
  [Vy] -> Add/1
  omega/1 -> Bus Selector/1
  Multiply2/1 -> Add1/2
  [delta_R] -> Minus/1
  [Vx] -> Add2/1
  [yaw_rate] -> Subsystem/1(In)
  Subsystem/1(Out) -> Add2/2
  [Vx] -> Add3/1
  [yaw_rate] -> Subsystem1/1(In)
  Subsystem1/1(Out) -> Add3/2
  Bus Selector/1 -> [yaw_rate]  "<yaw rate>"
  velocity limit1/1("velocity_limit ") -> Switch1/2
  [delta_L] -> Minus1/1
  Multiply3/1 -> Radians to Degrees1/1, alpha_fL/1
  velocity limit2/1("velocity_limit ") -> Switch3/2
  Radians to Degrees/1 -> [VD_alpha_fR]
  Radians to Degrees1/1 -> [VD_alpha_fL]

== system tadpole_dynamic_close_loop/Vehicle Model/Tadpole vehicle dynamic/Calculation/velocity limit1 ==
  note: let V>0.005 or V<-0.005, otherwise V = 0
  "velocity " : Inport
  If Action Subsystem2 : Subsystem  TreatAsAtomicUnit=on
  If Action Subsystem3 : Subsystem  TreatAsAtomicUnit=on
  If1 : If  IfExpression=u1>0
  Merge : Merge
  "velocity_limit " : Outport  VectorParamsAs1DForOutWhenUnconnected=off
  wires:
  Merge/1 -> "velocity_limit "/1
  "velocity "/1 -> If Action Subsystem3/1(In1), If Action Subsystem2/1(In1), If1/1
  If1/1 -> If Action Subsystem2/Action
  If1/2 -> If Action Subsystem3/Action
  If Action Subsystem2/1(Out1) -> Merge/1
  If Action Subsystem3/1(Out1) -> Merge/2

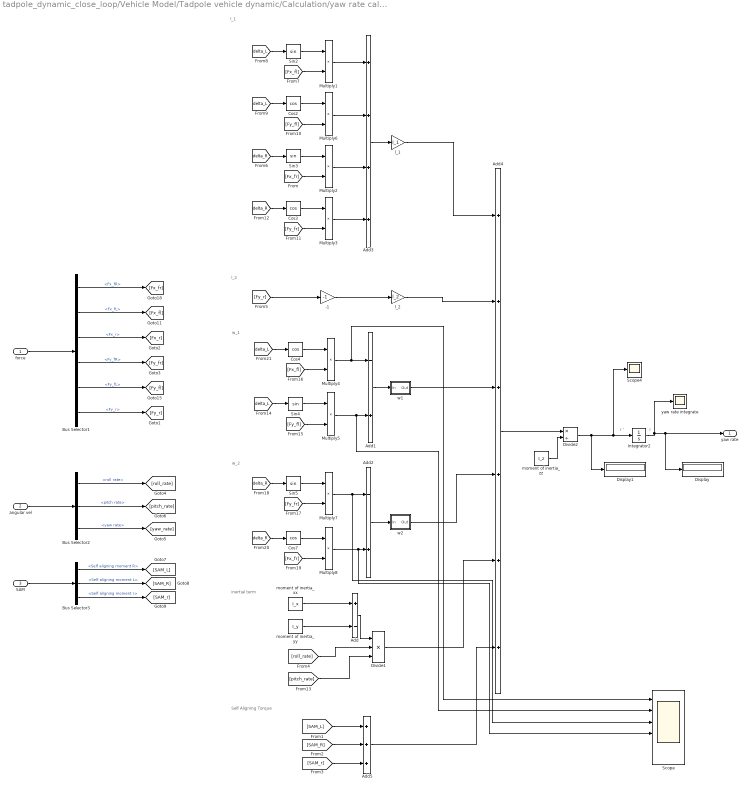
== system tadpole_dynamic_close_loop/Vehicle Model/Tadpole vehicle dynamic/Calculation/yaw rate calculation ==
  note: Self Aligning Torque
  note: inertial term
  note: w_2
  note: w_1
  note: l_2
  note: l_1
  note: r '
  note: r
  force : Inport
  angular vel : Inport  Port=2
  SAM : Inport  Port=3
  -1 : Gain  Gain=-1
  Add : Sum  Inputs=+-
  Add1 : Sum  Inputs=-+
  Add2 : Sum  Inputs=-+
  Add3 : Sum  Inputs=++++
  Add4 : Sum  Inputs=++++++
  Add5 : Sum  Inputs=+++
  Bus Selector1 : BusSelector  OutputSignals=Fx_fR,Fx_fL,Fx_r,Fy_fR,Fy_fL,Fy_r
  Bus Selector2 : BusSelector  OutputSignals=roll rate,pitch rate,yaw rate
  Bus Selector3 : BusSelector  OutputSignals=Self aligning moment R,Self aligning moment L,Self aligning moment r
  Cos{2..4,7} (4 alike) : Trigonometry  Operator=cos
  Display : Display
  Display1 : Display
  Divide1 : Product  Inputs=***
  Divide2 : Product  Inputs=*/
  Integrator2 : Integrator
  Multiply{1..8} (8 alike) : Product
  Scope : Scope  NumInputPorts=6
  Scope4 : Scope
  Sin{2..5} (4 alike) : Trigonometry
  l_1 : Gain  Gain=l_1
  l_2 : Gain  Gain=l_2
  moment of inertia_xx : Constant  Value=I_x
  moment of inertia_yy : Constant  Value=I_y
  moment of inertia_zz : Constant  Value=I_z
  w1 : Subsystem
  w2 : Subsystem
  yaw rate integrate : Scope
  yaw rate : Outport  VectorParamsAs1DForOutWhenUnconnected=off
  wires:
  force/1 -> Bus Selector1/1
  [delta_L] -> Sin2/1
  Sin2/1 -> Multiply1/1
  [Fx_fl] -> Multiply1/2
  [delta_L] -> Cos2/1
  Cos2/1 -> Multiply6/1
  [Fy_fl] -> Multiply6/2
  [Fx_fr] -> Multiply2/2
  [delta_R] -> Sin3/1
  Sin3/1 -> Multiply2/1
  [Fy_fr] -> Multiply3/2
  Cos3/1 -> Multiply3/1
  [delta_R] -> Cos3/1
  Multiply1/1 -> Add3/1
  Multiply6/1 -> Add3/2
  Multiply2/1 -> Add3/3
  Multiply3/1 -> Add3/4
  Add3/1 -> l_1/1
  -1/1 -> l_2/1
  [Fy_r] -> -1/1
  [delta_L] -> Cos4/1
  Cos4/1 -> Multiply4/1
  Multiply4/1 -> Scope/1, Add1/1
  [Fx_fl] -> Multiply4/2
  [Fy_fl] -> Multiply5/2
  Sin4/1 -> Multiply5/1
  [delta_L] -> Sin4/1
  [delta_R] -> Cos7/1
  Cos7/1 -> Multiply8/1
  [Fx_fr] -> Multiply8/2
  [Fy_fr] -> Multiply7/2
  Sin5/1 -> Multiply7/1
  [delta_R] -> Sin5/1
  Multiply5/1 -> Scope/2, Add1/2
  Multiply7/1 -> Scope/3, Add2/1
  Multiply8/1 -> Scope/4, Add2/2
  Add1/1 -> w1/1(In)
  Add2/1 -> w2/1(In)
  Divide2/1 -> Display1/1, Scope4/1, Integrator2/1
  moment of inertia_zz/1 -> Divide2/2
  Add4/1 -> Divide2/1
  l_1/1 -> Add4/1
  l_2/1 -> Add4/2
  w1/1(Out) -> Add4/3
  w2/1(Out) -> Add4/4
  Bus Selector1/1 -> [Fx_fr]  "<Fx_fR>"
  Bus Selector1/2 -> [Fx_fl]  "<Fx_fL>"
  Bus Selector1/3 -> [Fx_r]  "<Fx_r>"
  Bus Selector1/4 -> [Fy_fr]  "<Fy_fR>"
  Bus Selector1/5 -> [Fy_fl]  "<Fy_fL>"
  Bus Selector1/6 -> [Fy_r]  "<Fy_r>"
  angular vel/1 -> Bus Selector2/1
  Bus Selector2/1 -> [roll_rate]  "<roll rate>"
  Bus Selector2/2 -> [pitch_rate]  "<pitch rate>"
  Bus Selector2/3 -> [yaw_rate]  "<yaw rate>"
  SAM/1 -> Bus Selector3/1
  Bus Selector3/1 -> [SAM_L]  "<Self aligning moment R>"
  Bus Selector3/2 -> [SAM_R]  "<Self aligning moment L>"
  Bus Selector3/3 -> [SAM_r]  "<Self aligning moment r>"
  [SAM_r] -> Add5/3
  moment of inertia_xx/1 -> Add/1
  moment of inertia_yy/1 -> Add/2
  Add/1 -> Divide1/1
  [roll_rate] -> Divide1/2
  [pitch_rate] -> Divide1/3
  Divide1/1 -> Add4/5
  [SAM_L] -> Add5/1
  [SAM_R] -> Add5/2
  Add5/1 -> Add4/6
  Integrator2/1 -> Display/1, yaw rate/1, yaw rate integrate/1

== system tadpole_dynamic_close_loop/Vehicle Model/resistance calculation/Rear Traction add up/Fm<0 ==
  |break| : Inport
  |motor| : Inport  Port=2
  "velocity sign " : Inport  Port=3
  Action Port : ActionPort  ActionPortLabel=else
  Add : Sum
  Merge1 : Merge  Inputs=3
  Sign : Signum
  Subtract1 : Sum  Inputs=+-
  Switch Case Action Subsystem15 : Subsystem  TreatAsAtomicUnit=on
  Switch Case Action Subsystem6 : Subsystem  TreatAsAtomicUnit=on
  Switch Case Action Subsystem7 : Subsystem  TreatAsAtomicUnit=on
  Switch Case2 : SwitchCase  CaseConditions={1,-1}
  Out1 : Outport  VectorParamsAs1DForOutWhenUnconnected=off
  wires:
  Switch Case2/3 -> Switch Case Action Subsystem7/Action  "m=b"
  [v_sign_b] -> Switch Case Action Subsystem6/1("value ")
  Switch Case2/2 -> Switch Case Action Subsystem6/Action  "m<b"
  |motor|/1 -> Add/1, Subtract1/1
  Switch Case Action Subsystem15/1(Out1) -> Merge1/1
  [v_sign_b] -> Switch Case Action Subsystem15/1("value ")
  Merge1/1 -> Out1/1
  Switch Case Action Subsystem6/1(Out1) -> Merge1/2
  |break|/1 -> Add/2, Subtract1/2
  Switch Case2/1 -> Switch Case Action Subsystem15/Action
  Add/1 -> [add_b]
  [v_sign_b] -> Switch Case Action Subsystem7/1("value ")
  Switch Case Action Subsystem7/1(Out1) -> Merge1/3
  Subtract1/1 -> Sign/1, [minus_b]
  "velocity sign "/1 -> [v_sign_b]
  Sign/1 -> Switch Case2/1

== system tadpole_dynamic_close_loop/Vehicle Model/resistance calculation/Rear Traction add up/Fm>=0 ==
  |break| : Inport
  |motor| : Inport  Port=2
  "velocity sign " : Inport  Port=3
  Action Port : ActionPort  ActionPortLabel=if(u1 >= 0)
  Add : Sum
  Merge : Merge  Inputs=3
  Merge1 : Merge  Inputs=3
  Scope : Scope
  Scope1 : Scope
  Scope2 : Scope
  Sign : Signum
  Subtract : Sum  Inputs=+-
  Switch Case Action Subsystem6 : Subsystem  TreatAsAtomicUnit=on
  Switch Case Action Subsystem7 : Subsystem  TreatAsAtomicUnit=on
  Switch Case2 : SwitchCase  CaseConditions={1,-1}
  m>b : Subsystem  TreatAsAtomicUnit=on
  Out1 : Outport  VectorParamsAs1DForOutWhenUnconnected=off
  wires:
  m>b/1(Out1) -> Merge/1
  Switch Case Action Subsystem6/1(Out1) -> Merge/2
  Switch Case Action Subsystem7/1(Out1) -> Merge/3
  Merge/1 -> Scope2/1, Out1/1
  |motor|/1 -> Add/1, Subtract/1
  |break|/1 -> Add/2, Subtract/2
  Subtract/1 -> [minus], Sign/1, Scope/1
  Add/1 -> [add]
  Switch Case2/1 -> m>b/Action
  [v_sign] -> m>b/1("velocity sign ")
  [v_sign] -> Switch Case Action Subsystem6/1("value ")
  Switch Case2/2 -> Switch Case Action Subsystem6/Action  "m<b"
  [v_sign] -> Switch Case Action Subsystem7/1("value ")
  Switch Case2/3 -> Switch Case Action Subsystem7/Action  "m=b"
  "velocity sign "/1 -> [v_sign]
  [add] -> m>b/2(add)
  [minus] -> m>b/3("minus ")
  [add] -> Switch Case Action Subsystem6/2(In2)
  [minus] -> Switch Case Action Subsystem6/3(In3)
  [add] -> Switch Case Action Subsystem7/2(In2)
  [minus] -> Switch Case Action Subsystem7/3(In3)
  m>b/2(Out2) -> Merge1/1
  Switch Case Action Subsystem6/2(Out2) -> Merge1/2
  Switch Case Action Subsystem7/2(Out2) -> Merge1/3
  Merge1/1 -> Scope1/1
  Sign/1 -> Switch Case2/1

== system tadpole_dynamic_close_loop/Vehicle Model/resistance calculation/Rolling Resistance Force Front L/Subsystem ==
  Vx : Inport
  Vy : Inport  Port=2
  yaw rate : Inport  Port=3
  Delta_L : Inport  Port=4
  Add : Sum  Inputs=+-
  Add1 : Sum
  Add2 : Sum
  Cos : Trigonometry  Operator=cos
  Cos1 : Trigonometry
  Gain1 : Gain  Gain=l_1
  Product : Product
  Product1 : Product
  w_1 : Subsystem
  Vx_Wheel : Outport  VectorParamsAs1DForOutWhenUnconnected=off
  wires:
  Delta_L/1 -> Cos1/1, Cos/1
  Cos/1 -> Product/1
  Vx/1 -> Add/1
  w_1/1(Out) -> Add/2
  yaw rate/1 -> w_1/1(In), Gain1/1
  Vy/1 -> Add1/2
  Gain1/1 -> Add1/1
  Add/1 -> Product/2
  Cos1/1 -> Product1/1
  Add1/1 -> Product1/2
  Product/1 -> Add2/1
  Product1/1 -> Add2/2
  Add2/1 -> Vx_Wheel/1

== system tadpole_dynamic_close_loop/Vehicle Model/resistance calculation/Rolling Resistance Force Front L/mu(v) ==
  Vx : Inport
  Add : Sum
  Constant : Constant  Value=mu_rolling_1
  Constant1 : Constant  Value=mu_rolling_2
  Product : Product
  Square : Math  Operator=square  SaturateOnIntegerOverflow=on
  mu_rolling : Outport  VectorParamsAs1DForOutWhenUnconnected=off
  tag scope: frct_roll_coe_fL=global
  wires:
  Constant/1 -> Add/1
  Constant1/1 -> Product/1
  Vx/1 -> Square/1
  Square/1 -> Product/2
  Add/1 -> [frct_roll_coe_fL], mu_rolling/1
  Product/1 -> Add/2

== system tadpole_dynamic_close_loop/Vehicle Model/resistance calculation/Rolling Resistance Force Front R/Subsystem ==
  Vx : Inport
  Vy : Inport  Port=2
  yaw rate : Inport  Port=3
  Delta_R : Inport  Port=4
  Add : Sum
  Add1 : Sum
  Add2 : Sum
  Cos : Trigonometry  Operator=cos
  Cos1 : Trigonometry
  Gain1 : Gain  Gain=l_1
  Product : Product
  Product1 : Product
  w_2 : Subsystem
  Vx_Wheel : Outport  VectorParamsAs1DForOutWhenUnconnected=off
  wires:
  Delta_R/1 -> Cos1/1, Cos/1
  Cos/1 -> Product/1
  Vx/1 -> Add/1
  w_2/1(Out) -> Add/2
  yaw rate/1 -> w_2/1(In), Gain1/1
  Vy/1 -> Add1/2
  Gain1/1 -> Add1/1
  Add/1 -> Product/2
  Cos1/1 -> Product1/1
  Add1/1 -> Product1/2
  Product/1 -> Add2/1
  Product1/1 -> Add2/2
  Add2/1 -> Vx_Wheel/1

== system tadpole_dynamic_close_loop/Vehicle Model/resistance calculation/Rolling Resistance Force Front R/mu(v) ==
  Vx : Inport
  Add : Sum
  Constant : Constant  Value=mu_rolling_1
  Constant1 : Constant  Value=mu_rolling_2
  Product : Product
  Square : Math  Operator=square  SaturateOnIntegerOverflow=on
  mu_rolling : Outport  VectorParamsAs1DForOutWhenUnconnected=off
  tag scope: frct_roll_coe_fR=global
  wires:
  Constant/1 -> Add/1
  Constant1/1 -> Product/1
  Vx/1 -> Square/1
  Square/1 -> Product/2
  Add/1 -> [frct_roll_coe_fR], mu_rolling/1
  Product/1 -> Add/2

== system tadpole_dynamic_close_loop/Vehicle Model/resistance calculation/Rolling Resistance Force Rear/mu(v) ==
  Vx : Inport
  Add : Sum
  Constant : Constant  Value=mu_rolling_1
  Constant1 : Constant  Value=mu_rolling_2
  Product : Product
  Square : Math  Operator=square  SaturateOnIntegerOverflow=on
  mu_rolling : Outport  VectorParamsAs1DForOutWhenUnconnected=off
  tag scope: frct_roll_coe_r=global
  wires:
  Constant/1 -> Add/1
  Constant1/1 -> Product/1
  Vx/1 -> Square/1
  Square/1 -> Product/2
  Add/1 -> [frct_roll_coe_r], mu_rolling/1
  Product/1 -> Add/2

== system tadpole_dynamic_close_loop/Vehicle Model/resistance calculation/linear slip cal. /slip recgonition ==
  In2 : Inport
  In3 : Inport  Port=2
  Constant : Constant
  Constant1 : Constant  Value=-1
  Display : Display
  If : If  IfExpression=u1~=0
  If Action Subsystem : Subsystem  TreatAsAtomicUnit=on
  If Action Subsystem1 : Subsystem  TreatAsAtomicUnit=on
  Merge : Merge
  Subtract : Sum  Inputs=+-
  tag scope: DBW_drive_slip_reg=global
  wires:
  Constant/1 -> If Action Subsystem/1(In1)
  If/1 -> If Action Subsystem/Action
  Subtract/1 -> If/1
  If Action Subsystem/1(Out1) -> Merge/1
  In2/1 -> Subtract/1
  If/2 -> If Action Subsystem1/Action
  In3/1 -> Subtract/2
  If Action Subsystem1/1(Out1) -> Merge/2
  Constant1/1 -> If Action Subsystem1/1(In1)
  Merge/1 -> Display/1, [DBW_drive_slip_reg]

== system tadpole_dynamic_close_loop/Vehicle Model/resistance calculation/velocity limit x/If Action Subsystem2 ==
  In1 : Inport
  Action Port : ActionPort  ActionPortLabel=if(u1>0 )
  Constant : Constant  Value=0
  If : If  IfExpression=0.005>u1
  If Action Subsystem : Subsystem  TreatAsAtomicUnit=on
  If Action Subsystem1 : Subsystem  TreatAsAtomicUnit=on
  Merge : Merge
  Out1 : Outport  VectorParamsAs1DForOutWhenUnconnected=off
  wires:
  Merge/1 -> Out1/1
  If Action Subsystem1/1(Out1) -> Merge/2
  If Action Subsystem/1(Out1) -> Merge/1
  Constant/1 -> If Action Subsystem/1(In1)
  If/2 -> If Action Subsystem1/Action
  If/1 -> If Action Subsystem/Action
  In1/1 -> If Action Subsystem1/1(In1), If/1

== system tadpole_dynamic_close_loop/Vehicle Model/resistance calculation/velocity limit x/If Action Subsystem3 ==
  In1 : Inport
  Action Port : ActionPort  ActionPortLabel=else
  Constant : Constant  Value=0
  If : If  IfExpression=-0.005<u1
  If Action Subsystem : Subsystem  TreatAsAtomicUnit=on
  If Action Subsystem1 : Subsystem  TreatAsAtomicUnit=on
  Merge : Merge
  Out1 : Outport  VectorParamsAs1DForOutWhenUnconnected=off
  wires:
  In1/1 -> If Action Subsystem1/1(In1), If/1
  If/1 -> If Action Subsystem/Action
  If/2 -> If Action Subsystem1/Action
  Constant/1 -> If Action Subsystem/1(In1)
  If Action Subsystem/1(Out1) -> Merge/1
  If Action Subsystem1/1(Out1) -> Merge/2
  Merge/1 -> Out1/1

== system tadpole_dynamic_close_loop/Vehicle Model/resistance calculation/velocity limit y/If Action Subsystem2 ==
  In1 : Inport
  Action Port : ActionPort  ActionPortLabel=if(u1>0 )
  Constant : Constant  Value=0
  If : If  IfExpression=0.005>u1
  If Action Subsystem : Subsystem  TreatAsAtomicUnit=on
  If Action Subsystem1 : Subsystem  TreatAsAtomicUnit=on
  Merge : Merge
  Out1 : Outport  VectorParamsAs1DForOutWhenUnconnected=off
  wires:
  Merge/1 -> Out1/1
  If Action Subsystem1/1(Out1) -> Merge/2
  If Action Subsystem/1(Out1) -> Merge/1
  Constant/1 -> If Action Subsystem/1(In1)
  If/2 -> If Action Subsystem1/Action
  If/1 -> If Action Subsystem/Action
  In1/1 -> If Action Subsystem1/1(In1), If/1

== system tadpole_dynamic_close_loop/Vehicle Model/resistance calculation/velocity limit y/If Action Subsystem3 ==
  In1 : Inport
  Action Port : ActionPort  ActionPortLabel=else
  Constant : Constant  Value=0
  If : If  IfExpression=-0.005<u1
  If Action Subsystem : Subsystem  TreatAsAtomicUnit=on
  If Action Subsystem1 : Subsystem  TreatAsAtomicUnit=on
  Merge : Merge
  Out1 : Outport  VectorParamsAs1DForOutWhenUnconnected=off
  wires:
  In1/1 -> If Action Subsystem1/1(In1), If/1
  If/1 -> If Action Subsystem/Action
  If/2 -> If Action Subsystem1/Action
  Constant/1 -> If Action Subsystem/1(In1)
  If Action Subsystem/1(Out1) -> Merge/1
  If Action Subsystem1/1(Out1) -> Merge/2
  Merge/1 -> Out1/1

== system tadpole_dynamic_close_loop/Vehicle Model/Tadpole vehicle dynamic/Calculation/Side slip angle Rear/velocity limit1 ==
  note: let V>0.0005 or V<-0.0005, otherwise V = 0
  "velocity " : Inport
  If Action Subsystem2 : Subsystem  TreatAsAtomicUnit=on
  If Action Subsystem3 : Subsystem  TreatAsAtomicUnit=on
  If1 : If  IfExpression=u1>0
  Merge : Merge
  "velocity_limit " : Outport  VectorParamsAs1DForOutWhenUnconnected=off
  wires:
  Merge/1 -> "velocity_limit "/1
  "velocity "/1 -> If Action Subsystem3/1(In1), If Action Subsystem2/1(In1), If1/1
  If1/1 -> If Action Subsystem2/Action
  If1/2 -> If Action Subsystem3/Action
  If Action Subsystem2/1(Out1) -> Merge/1
  If Action Subsystem3/1(Out1) -> Merge/2

== system tadpole_dynamic_close_loop/Vehicle Model/Tadpole vehicle dynamic/Calculation/Subsystem1/Subsystem ==
  Fy_fR : Inport
  "linear slip cal fR " : Subsystem
  Lateral force fR : Outport  VectorParamsAs1DForOutWhenUnconnected=off
  wires:
  [Force_Fz_fR] -> "linear slip cal fR "/2(Normal Force)
  "linear slip cal fR "/1(Lateral force) -> Lateral force fR/1
  Fy_fR/1 -> "linear slip cal fR "/1(Lateral Force)

== system tadpole_dynamic_close_loop/Vehicle Model/Tadpole vehicle dynamic/Calculation/Subsystem1/velocity limit ==
  "velocity " : Inport
  If Action Subsystem2 : Subsystem  TreatAsAtomicUnit=on
  If Action Subsystem3 : Subsystem  TreatAsAtomicUnit=on
  If1 : If  IfExpression=u1>0
  Merge : Merge
  "velocity_limit " : Outport  VectorParamsAs1DForOutWhenUnconnected=off
  wires:
  Merge/1 -> "velocity_limit "/1
  "velocity "/1 -> If Action Subsystem3/1(In1), If Action Subsystem2/1(In1), If1/1
  If1/1 -> If Action Subsystem2/Action
  If1/2 -> If Action Subsystem3/Action
  If Action Subsystem2/1(Out1) -> Merge/1
  If Action Subsystem3/1(Out1) -> Merge/2

== system tadpole_dynamic_close_loop/Vehicle Model/Tadpole vehicle dynamic/Calculation/Subsystem2/Subsystem ==
  Fy_fL : Inport
  "linear slip cal r " : Subsystem
  Lateral Force r : Outport  VectorParamsAs1DForOutWhenUnconnected=off
  wires:
  [Force_Fz_r] -> "linear slip cal r "/2(Normal Force)
  "linear slip cal r "/1(Lateral force) -> Lateral Force r/1
  Fy_fL/1 -> "linear slip cal r "/1(Lateral Force)

== system tadpole_dynamic_close_loop/Vehicle Model/Tadpole vehicle dynamic/Calculation/Subsystem2/velocity limit ==
  "velocity " : Inport
  If Action Subsystem2 : Subsystem  TreatAsAtomicUnit=on
  If Action Subsystem3 : Subsystem  TreatAsAtomicUnit=on
  If1 : If  IfExpression=u1>0
  Merge : Merge
  "velocity_limit " : Outport  VectorParamsAs1DForOutWhenUnconnected=off
  wires:
  Merge/1 -> "velocity_limit "/1
  "velocity "/1 -> If Action Subsystem3/1(In1), If Action Subsystem2/1(In1), If1/1
  If1/1 -> If Action Subsystem2/Action
  If1/2 -> If Action Subsystem3/Action
  If Action Subsystem2/1(Out1) -> Merge/1
  If Action Subsystem3/1(Out1) -> Merge/2

== system tadpole_dynamic_close_loop/Vehicle Model/Tadpole vehicle dynamic/Calculation/Subsystem3/Subsystem ==
  Fy_fL : Inport
  "linear slip cal fL " : Subsystem
  Lateral Force fL : Outport  VectorParamsAs1DForOutWhenUnconnected=off
  wires:
  [Force_Fz_fL] -> "linear slip cal fL "/2(Normal Force)
  "linear slip cal fL "/1(Lateral force) -> Lateral Force fL/1
  Fy_fL/1 -> "linear slip cal fL "/1(Lateral Force)

== system tadpole_dynamic_close_loop/Vehicle Model/Tadpole vehicle dynamic/Calculation/Subsystem3/velocity limit ==
  "velocity " : Inport
  If Action Subsystem2 : Subsystem  TreatAsAtomicUnit=on
  If Action Subsystem3 : Subsystem  TreatAsAtomicUnit=on
  If1 : If  IfExpression=u1>0
  Merge : Merge
  "velocity_limit " : Outport  VectorParamsAs1DForOutWhenUnconnected=off
  wires:
  Merge/1 -> "velocity_limit "/1
  "velocity "/1 -> If Action Subsystem3/1(In1), If Action Subsystem2/1(In1), If1/1
  If1/1 -> If Action Subsystem2/Action
  If1/2 -> If Action Subsystem3/Action
  If Action Subsystem2/1(Out1) -> Merge/1
  If Action Subsystem3/1(Out1) -> Merge/2

== system tadpole_dynamic_close_loop/Vehicle Model/Tadpole vehicle dynamic/Calculation/Velocity x/Equivalent mass ==
  Add1 : Sum  Inputs=+++
  Constant : Constant  Value=2
  Divide1 : Product  Inputs=*/*
  Divide2 : Product  Inputs=*/
  Initial wheel radius : Constant  Value=R_0
  Square : Math  Operator=square  SignedPower=off  SaturateOnIntegerOverflow=on
  Square1 : Math  Operator=square  SignedPower=off  SaturateOnIntegerOverflow=on
  front wheel mass inertial : Constant  Value=I_f_wheel
  mass of vehicle : Constant  Value=m
  rear wheel mass inertial : Constant  Value=I_r_wheel
  Mass_eq : Outport  VectorParamsAs1DForOutWhenUnconnected=off
  wires:
  Divide2/1 -> Add1/3
  Add1/1 -> Mass_eq/1
  Divide1/1 -> Add1/2
  [R_h] -> Square/1
  Initial wheel radius/1 -> Square1/1
  rear wheel mass inertial/1 -> Divide2/1
  mass of vehicle/1 -> Add1/1
  front wheel mass inertial/1 -> Divide1/1
  Square/1 -> Divide1/2
  Square1/1 -> Divide2/2
  Constant/1 -> Divide1/3

== system tadpole_dynamic_close_loop/Vehicle Model/Tadpole vehicle dynamic/Calculation/side slip angle Front/Subsystem ==
  In : Inport
  Product : Product
  Out : Outport  VectorParamsAs1DForOutWhenUnconnected=off
  wires:
  [w_1] -> Product/2
  Product/1 -> Out/1
  In/1 -> Product/1

== system tadpole_dynamic_close_loop/Vehicle Model/Tadpole vehicle dynamic/Calculation/side slip angle Front/Subsystem1 ==
  In : Inport
  Product : Product
  Out : Outport  VectorParamsAs1DForOutWhenUnconnected=off
  wires:
  [w_2] -> Product/2
  Product/1 -> Out/1
  In/1 -> Product/1
